simulink model "BlockV5"  (R2017a)
settings: Solver=VariableStepAuto  StartTime=0.0  StopTime=Tsim  FixedStep=Ts_compute  RelTol=1e-3
values from neighbouring files (symbols this model uses):
  A = [0 ur2 0;-ur2 0 ur1;0 0 0]    [Model_old.m]    (also in PIController.m)
  b = 0.1    [Model_old.m]
  C = eye(3)    [Model_old.m]    (also in PIController.m)
  g = 40    [Model_old.m]    (also in ModeloBase_OLD.m)
  J = 0.01    [Model_old.m]
  Kd = 0    [Model_old.m]
  Ke = 0.08    [Model_old.m]
  Ki = 10.0    (= 10)    [Model_old.m]
  Kp = 5.0    (= 5)    [Model_old.m]
  ksi = 0.6    [Model_old.m]    (also in ModeloBase_OLD.m = 0.3)
  L = 0.5    [Model_old.m]
  R = 1    [Model_old.m]
  Rv = var(noise.data)    [Model_old.m]
  Ts = 0.1    [Model_old.m]    (also in ModeloBase_OLD.m; PIController.m)
  Ts_sensor = 1/50    (= 0.02)    [Model_old.m]
undefined symbols (not defined in the file or in its folder): Ad, DiscIntNeverNeededParam, F_M, Rw, Ts_compute, Vd
libraries: simulink x26, cstblocks x6, simulink_extras x2
settings Model: PauseTimes=28  NumberOfSteps=10  Creator=davi2  LastModifiedBy=davi2

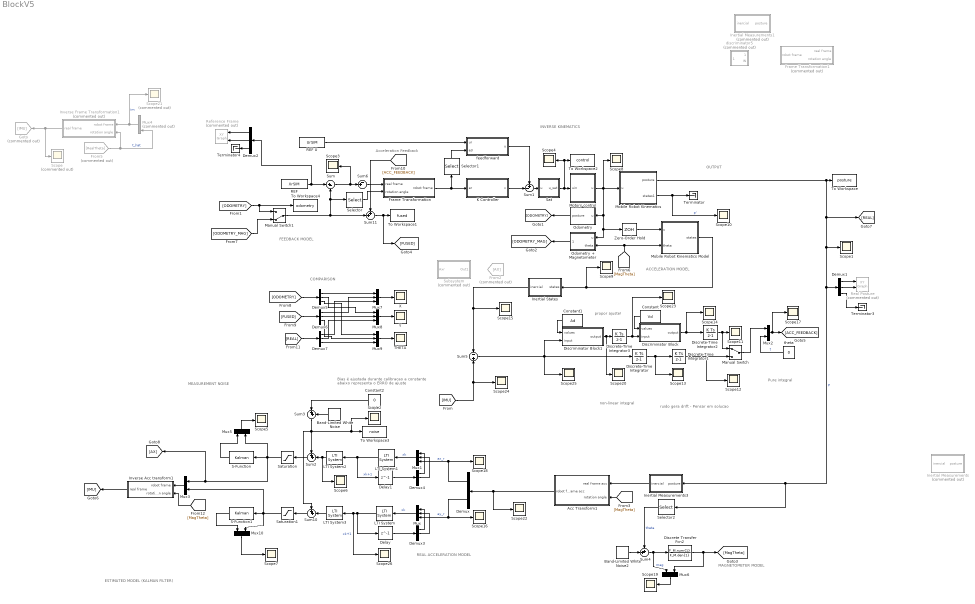
== system BlockV5 ==
  note: COMPARISON
  note: Bias é ajustada durante calibracao
      | a constante abaixo representa o ERRO de ajuste
  note: propor ajuste!
  note: Pure integral
  note: Acceleration Feedback
  note: ACCELERATION MODEL
  note: ruido gera drift - Pensar em solucao
  note: OUTPUT
  note: MEASUREMENT NOISE
  note: REAL ACCELERATION
      | MODEL
  note: INVERSE KINEMATICS
  note: MAGNETOMETER MODEL
  note: FEEDBACK MODEL
  note: ESTIMATED MODEL (KALMAN FILTER)
  note: non-linear integral
  Acc Transform1 : Subsystem
  Band-Limited White Noise : simulink/Sources/Band-Limited White Noise  Cov=0.00001  Ts=Ts_sensor  seed=[23341]
  Band-Limited White Noise2 : simulink/Sources/Band-Limited White Noise  Cov=0.00001  Ts=1/200  seed=[23341]
  Constant : Constant  Value=Vd
  Constant1 : Constant  Value=Ad
  Constant2 : Constant  Value=0
  Delay : Delay  DelayLength=1
  Delay1 : Delay  DelayLength=1
  Demux : Demux  Outputs=2
  Demux{1..7} (7 alike) : Demux  Outputs=3
  Discrete Transfer Fcn2 : DiscreteTransferFcn  Numerator=F_M.num{1}  Denominator=F_M.den{1}  SampleTime=Ts_sensor
  Discrete-Time Integrator{,1..3} (4 alike) : DiscreteIntegrator  InitialConditionSetting=State (most efficient)  SampleTime=Ts_sensor  ICPrevOutput=DiscIntNeverNeededParam  ICPrevScaledInput=DiscIntNeverNeededParam
  Discriminator Block : Subsystem
  Discriminator Block1 : Subsystem
  Frame Transformation : Subsystem
  Frame Transformation1 : Subsystem  Commented=on
  From2 : From  Commented=on  GotoTag=AX
  From5 : From  Commented=on  GotoTag=RealTheta
  Goto : Goto  Commented=on  GotoTag=IMU
  Inertial Measurements : Subsystem  Commented=on
  Inertial Measurements1 : Subsystem  Commented=on
  Inertial Measurements3 : Subsystem
  Inertial States : Subsystem
  Inverse Acc transform1 : Subsystem
  Inverse Frame Transformation1 : Subsystem  Commented=on
  K Controller : Subsystem
  LTI System : cstblocks/LTI System  sys=A  IC=[]
  LTI System1 : cstblocks/LTI System  sys=A  IC=[]
  LTI System2 : cstblocks/LTI System  sys=C  IC=[]
  LTI System3 : cstblocks/LTI System  sys=C  IC=[]
  Manual Switch : ManualSwitch
  Manual Switch1 : ManualSwitch  CurrentSetting=0
  Mobile Robot Kinematics : Subsystem
  Mobile Robot Kinematics Model : Subsystem
  Motors control : Subsystem
  Mux{,1,7..9} (5 alike) : Mux  Inputs=3
  Mux{2..3,5..6,10} (5 alike) : Mux  Inputs=2
  Mux4 : Mux  Commented=on  Inputs=3
  Odometry : Subsystem
  Odometry + Magnetometer : Subsystem
  REF : FromWorkspace  VariableName=XrSIM  SampleTime=Ts  OutputAfterFinalValue=Holding final value
  REF U : FromWorkspace  VariableName=UrSIM  SampleTime=Ts  OutputAfterFinalValue=Holding final value
  Real Posture : simulink/Sinks/XY Graph  Commented=on  xmin=0  xmax=3  ymin=-0.8  ymax=1.5  st=Ts
  Reference Frame : simulink/Sinks/XY Graph  Commented=on  xmin=0  xmax=2  ymin=0  ymax=1.5  st=Ts
  S-Function : S-Function  FunctionName=Kalman  Parameters=Ts_sensor,A,C,Rw,Rv  SFunctionDeploymentMode=off  EnableBusSupport=off
  S-Function1 : S-Function  FunctionName=Kalman  Parameters=Ts_sensor,A,C,Rw,Rv  SFunctionDeploymentMode=off  EnableBusSupport=off
  Sat : Subsystem
  Saturation : Saturate  UpperLimit=4*9.8  LowerLimit=-4*9.8
  Saturation1 : Saturate  UpperLimit=4*9.8  LowerLimit=-4*9.8
  Scope : Scope  Commented=on
  Scope{1..20,22..26} (25 alike) : Scope
  Scope21 : Scope  Commented=on
  Selector : Selector  InputPortWidth=3  IndexOptions=Index vector (dialog)  Indices=3  OutputSizes=1
  Selector1 : Selector  InputPortWidth=3  IndexOptions=Index vector (dialog)  Indices=3  OutputSizes=1
  Selector2 : Selector  InputPortWidth=3  IndexOptions=Index vector (dialog)  Indices=3  OutputSizes=1
  Subsystem : Subsystem  Commented=on
  Sum : Sum  Inputs=|+-
  Sum1 : Sum  Inputs=+-|
  Sum{2,4,10..11} (4 alike) : Sum  Inputs=++|
  Sum3 : Sum  Inputs=|++
  Sum5 : Sum  Inputs=-+
  Sum6 : Sum  Inputs=-+|
  THETA : Scope
  Terminator : Terminator
  Terminator3 : Terminator
  Terminator4 : Terminator
  To Workspace : ToWorkspace  VariableName=posture  SaveFormat=Timeseries  SampleTime=-1
  To Workspace1 : ToWorkspace  VariableName=fused  SaveFormat=Timeseries  SampleTime=-1
  To Workspace2 : ToWorkspace  VariableName=control  SaveFormat=Timeseries  SampleTime=-1
  To Workspace3 : ToWorkspace  VariableName=noise  SaveFormat=Timeseries  SampleTime=-1
  To Workspace4 : ToWorkspace  VariableName=odometry  SaveFormat=Timeseries  SampleTime=-1
  X : Scope
  Y : Scope
  Zero-Order Hold : ZeroOrderHold  SampleTime=Ts_sensor
  discriminator5 : Subsystem  Commented=on
  feedforward : Subsystem
  theta : Constant  Value=0
  wires:
  Sum/1 -> Sum6/2, Scope3/1
  Frame Transformation/1(robot frame) -> K Controller/1(er), Selector1/1
  REF U/1 -> feedforward/1(ur)
  Selector1/1 -> feedforward/2(e3)
  feedforward/1(u) -> Sum1/1
  K Controller/1(v) -> Sum1/2
  Motors control/1(u) -> Zero-Order Hold/1, Odometry + Magnetometer/1(u), Odometry/1(u), Mobile Robot Kinematics/1(u), Scope8/1
  Selector2/1 -> Sum4/1  "theta"
  Demux1/1 -> Real Posture/1
  Demux1/2 -> Real Posture/2
  REF/1 -> Demux2/1, Sum/1
  Odometry/1(posture) -> [ODOMETRY]
  Sum1/1 -> Sat/1(u)
  Sat/1(u_sat) -> Motors control/1(uin), Scope4/1, To Workspace2/1
  Demux1/3 -> Terminator3/1
  Band-Limited White Noise2/1 -> Sum4/2
  Sum4/1 -> Discrete Transfer Fcn2/1, Mux6/1  "mag"
  Discrete Transfer Fcn2/1 -> [MagTheta], Mux6/2
  Demux2/1 -> Reference Frame/1
  Demux2/2 -> Reference Frame/2
  Demux2/3 -> Terminator4/1
  LTI System/1 -> Scope26/1, LTI System3/1, Delay/1  "xk+1"
  Delay/1 -> Demux3/1
  Demux3/1 -> Mux/1
  Demux3/2 -> Mux/2
  Mux/1 -> LTI System/1  "xk"
  Demux4/2 -> Mux1/2
  Delay1/1 -> Demux4/1
  Demux4/1 -> Mux1/1
  LTI System1/1 -> Delay1/1, LTI System2/1  "xk+1"
  Mux1/1 -> LTI System1/1  "xk"
  Inverse Frame Transformation1/1(real frame) -> Goto/1, Scope/1
  From5/1 -> Mux4/3, Inverse Frame Transformation1/2(rotation angle)  "t_hat"
  LTI System3/1 -> Sum10/2
  Mux4/1 -> Scope21/1, Inverse Frame Transformation1/1(robot frame)  "im"
  Mobile Robot Kinematics/1(posture) -> [REAL], Selector2/1, Inertial Measurements3/1(posture), Demux1/1, Scope1/1, To Workspace/1  "P"
  Demux/1 -> Mux1/3, Scope18/1  "ax_r"
  Demux/2 -> Scope16/1, Mux/3  "ay_r"
  Inertial States/1(inercial) -> Sum5/1, Scope15/1
  Inertial Measurements3/1(inercial) -> Acc Transform1/1(real frame acc)
  Acc Transform1/1(robot frame acc) -> Scope22/1, Demux/1
  Sum6/1 -> Frame Transformation/1(real frame)
  theta/1 -> Mux2/2  "t"
  Mux2/1 -> Scope17/1, [ACC_FEEDBACK]
  LTI System2/1 -> Scope6/1, Sum2/2
  Sum11/1 -> [FUSED], To Workspace1/1
  Discrete-Time Integrator/1 -> Discrete-Time Integrator1/1, Scope13/1
  Mux5/1 -> Scope5/1
  Discrete-Time Integrator2/1 -> Scope11/1, Manual Switch/1
  Discrete-Time Integrator1/1 -> Manual Switch/2, Scope12/1
  Manual Switch/1 -> Mux2/1
  Discriminator Block/1(output) -> Discrete-Time Integrator2/1, Scope14/1
  Discriminator Block1/1(output) -> Scope20/1, Discrete-Time Integrator3/1
  Discrete-Time Integrator3/1 -> Discriminator Block/2(input), Scope23/1
  Constant1/1 -> Discriminator Block1/1(values)
  [ACC_FEEDBACK] -> Sum11/1
  Selector/1 -> Frame Transformation/2(rotation angle)
  [MagTheta] -> Acc Transform1/2(rotation angle)
  Odometry + Magnetometer/1(posture) -> [ODOMETRY_MAG]
  [MagTheta] -> Mobile Robot Kinematics Model/2("theta "), Odometry + Magnetometer/2(theta)
  [ODOMETRY] -> Manual Switch1/1, To Workspace4/1
  [ODOMETRY_MAG] -> Manual Switch1/2
  Manual Switch1/1 -> Selector/1, Sum/2, Sum11/2
  Mux6/1 -> Scope19/1
  [IMU] -> Scope24/1, Sum5/2
  [ODOMETRY] -> Demux5/1
  [FUSED] -> Demux6/1
  [REAL] -> Demux7/1
  Demux5/1 -> Mux7/1
  Demux6/1 -> Mux7/2
  Demux7/1 -> Mux7/3
  Mux7/1 -> X/1
  Demux5/2 -> Mux8/1
  Demux6/2 -> Mux8/2
  Demux7/2 -> Mux8/3
  Demux5/3 -> Mux9/1
  Demux6/3 -> Mux9/2
  Demux7/3 -> Mux9/3
  Mux8/1 -> Y/1
  Mux9/1 -> THETA/1
  Zero-Order Hold/1 -> Mobile Robot Kinematics Model/1(u)
  Mobile Robot Kinematics/2(states1) -> Scope10/1, Terminator/1  "p'"
  Mux3/1 -> Inverse Acc transform1/1(robot frame)
  [MagTheta] -> Inverse Acc transform1/2(rotation angle)
  Inverse Acc transform1/1(real frame) -> [IMU]
  Constant/1 -> Discriminator Block/1(values)
  Sum3/1 -> Sum10/1, Sum2/1, Scope2/1, To Workspace3/1
  Band-Limited White Noise/1 -> Sum3/2
  Constant2/1 -> Sum3/1
  Sum10/1 -> Saturation1/1
  Sum2/1 -> Saturation/1
  Sum5/1 -> Scope25/1, Discrete-Time Integrator/1, Discriminator Block1/2(input)
  Saturation1/1 -> Mux3/2, Mux10/2, S-Function1/1
  Saturation/1 -> [AX], Mux3/1, Mux5/2, S-Function/1
  S-Function1/1 -> Mux10/1
  Mux10/1 -> Scope7/1
  S-Function/1 -> Mux5/1
  Mobile Robot Kinematics Model/1(states) -> Scope9/1, Inertial States/1(states)

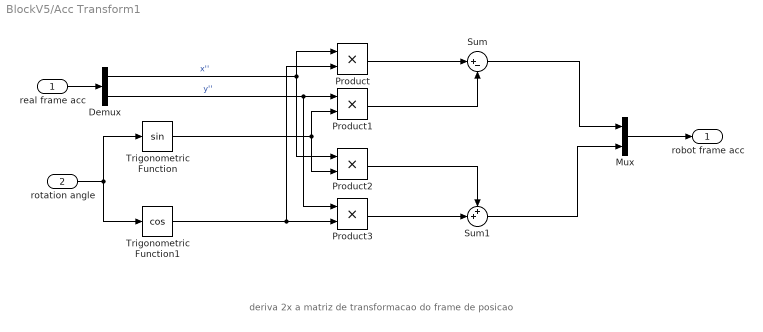
== system BlockV5/Acc Transform1 ==
  note: deriva 2x a matriz de transformacao do frame de posicao
  real frame acc : Inport
  rotation angle : Inport  Port=2
  Demux : Demux  Outputs=2
  Mux : Mux  Inputs=2
  Product{,1..3} (4 alike) : Product
  Sum : Sum  Inputs=|+-
  Sum1 : Sum  Inputs=++|
  Trigonometric Function : Trigonometry
  Trigonometric Function1 : Trigonometry  Operator=cos
  robot frame acc : Outport
  wires:
  rotation angle/1 -> Trigonometric Function/1, Trigonometric Function1/1
  Mux/1 -> robot frame acc/1
  real frame acc/1 -> Demux/1
  Demux/1 -> Product2/1, Product/1  "x''"
  Trigonometric Function1/1 -> Product/2, Product3/2
  Product/1 -> Sum/1
  Trigonometric Function/1 -> Product1/2, Product2/2
  Demux/2 -> Product3/1, Product1/1  "y''"
  Product1/1 -> Sum/2
  Sum/1 -> Mux/1
  Product3/1 -> Sum1/2
  Product2/1 -> Sum1/1
  Sum1/1 -> Mux/2

== system BlockV5/Discriminator Block ==
  values : Inport
  input : Inport  Port=2
  Demux : Demux  Outputs=2
  Mux : Mux  Inputs=2
  discriminator1 : Subsystem
  discriminator3 : Subsystem
  output : Outport
  wires:
  input/1 -> Demux/1
  Demux/1 -> discriminator3/2(IN)
  Demux/2 -> discriminator1/2(IN)
  Mux/1 -> output/1
  discriminator3/1(OUT) -> Mux/1
  discriminator1/1(OUT) -> Mux/2
  values/1 -> discriminator1/1(value), discriminator3/1(value)

== system BlockV5/Discriminator Block1 ==
  values : Inport
  input : Inport  Port=2
  Demux : Demux  Outputs=2
  Mux : Mux  Inputs=2
  discriminator1 : Subsystem
  discriminator3 : Subsystem
  output : Outport
  wires:
  input/1 -> Demux/1
  Demux/1 -> discriminator3/2(IN)
  Demux/2 -> discriminator1/2(IN)
  Mux/1 -> output/1
  discriminator3/1(OUT) -> Mux/1
  discriminator1/1(OUT) -> Mux/2
  values/1 -> discriminator1/1(value), discriminator3/1(value)

== system BlockV5/Frame Transformation ==
  real frame : Inport
  rotation angle : Inport  Port=2
  Mux : Mux  Inputs=2
  S-Function : S-Function  FunctionName=Real2Robot  Parameters=Ts  SFunctionDeploymentMode=off  EnableBusSupport=off
  robot frame : Outport
  wires:
  real frame/1 -> Mux/1
  rotation angle/1 -> Mux/2
  Mux/1 -> S-Function/1
  S-Function/1 -> robot frame/1

== system BlockV5/Frame Transformation1 ==
  real frame : Inport
  rotation angle : Inport  Port=2
  Mux : Mux  Inputs=2
  S-Function : S-Function  FunctionName=Real2Robot  Parameters=Ts_compute  SFunctionDeploymentMode=off  EnableBusSupport=off
  robot frame : Outport
  wires:
  real frame/1 -> Mux/1
  rotation angle/1 -> Mux/2
  Mux/1 -> S-Function/1
  S-Function/1 -> robot frame/1

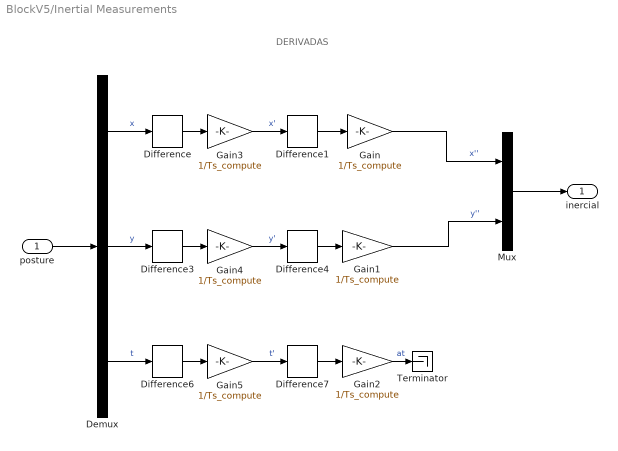
== system BlockV5/Inertial Measurements ==
  note: DERIVADAS
  posture : Inport
  Demux : Demux  Outputs=3
  Difference{,1,3..4,6..7} (6 alike) : simulink/Discrete/Difference  ICPrevInput=0.0  OutMin=[]  OutMax=[]  OutDataType=fixdt(1, 16)  OutScaling=2^-10  DoSatur=off
  Gain{,1..5} (6 alike) : Gain  Gain=1/Ts_compute
  Mux : Mux  Inputs=2
  Terminator : Terminator
  inercial : Outport
  wires:
  posture/1 -> Demux/1
  Demux/3 -> Difference6/1  "t"
  Demux/2 -> Difference3/1  "y"
  Demux/1 -> Difference/1  "x"
  Difference1/1 -> Gain/1
  Difference4/1 -> Gain1/1
  Difference7/1 -> Gain2/1
  Mux/1 -> inercial/1
  Gain2/1 -> Terminator/1  "at"
  Difference/1 -> Gain3/1
  Gain3/1 -> Difference1/1  "x'"
  Difference3/1 -> Gain4/1
  Gain4/1 -> Difference4/1  "y'"
  Difference6/1 -> Gain5/1
  Gain5/1 -> Difference7/1  "t'"
  Gain/1 -> Mux/1  "x''"
  Gain1/1 -> Mux/2  "y''"

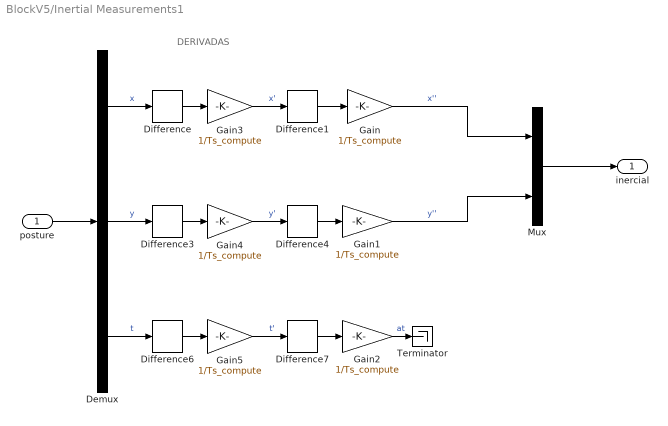
== system BlockV5/Inertial Measurements1 ==
  note: DERIVADAS
  posture : Inport
  Demux : Demux  Outputs=3
  Difference{,1,3..4,6..7} (6 alike) : simulink/Discrete/Difference  ICPrevInput=0.0  OutMin=[]  OutMax=[]  OutDataType=fixdt(1, 16)  OutScaling=2^-10  DoSatur=off
  Gain{,1..5} (6 alike) : Gain  Gain=1/Ts_compute
  Mux : Mux  Inputs=2
  Terminator : Terminator
  inercial : Outport
  wires:
  posture/1 -> Demux/1
  Demux/3 -> Difference6/1  "t"
  Demux/2 -> Difference3/1  "y"
  Demux/1 -> Difference/1  "x"
  Difference1/1 -> Gain/1
  Difference4/1 -> Gain1/1
  Difference7/1 -> Gain2/1
  Mux/1 -> inercial/1
  Gain2/1 -> Terminator/1  "at"
  Difference/1 -> Gain3/1
  Gain3/1 -> Difference1/1  "x'"
  Difference3/1 -> Gain4/1
  Gain4/1 -> Difference4/1  "y'"
  Difference6/1 -> Gain5/1
  Gain5/1 -> Difference7/1  "t'"
  Gain/1 -> Mux/1  "x''"
  Gain1/1 -> Mux/2  "y''"

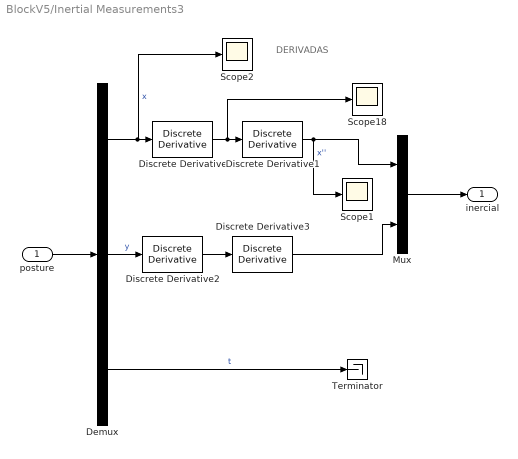
== system BlockV5/Inertial Measurements3 ==
  note: DERIVADAS
  posture : Inport
  Demux : Demux  Outputs=3
  Discrete Derivative{,1..3} (4 alike) : simulink/Discrete/Discrete Derivative  gainval=1.0  ICPrevScaledInput=0.0  OutMin=[]  OutMax=[]  OutDataType=fixdt(1, 16)  OutScaling=2^-10  DoSatur=off
  Mux : Mux  Inputs=2
  Scope1 : Scope
  Scope18 : Scope
  Scope2 : Scope
  Terminator : Terminator
  inercial : Outport
  wires:
  posture/1 -> Demux/1
  Demux/1 -> Discrete Derivative/1, Scope2/1  "x"
  Mux/1 -> inercial/1
  Discrete Derivative1/1 -> Scope1/1, Mux/1  "x''"
  Discrete Derivative/1 -> Scope18/1, Discrete Derivative1/1
  Demux/2 -> Discrete Derivative2/1  "y"
  Discrete Derivative2/1 -> Discrete Derivative3/1
  Discrete Derivative3/1 -> Mux/2
  Demux/3 -> Terminator/1  "t"

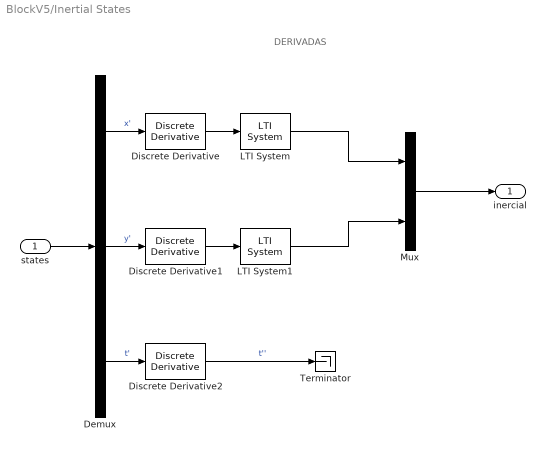
== system BlockV5/Inertial States ==
  note: DERIVADAS
  states : Inport
  Demux : Demux  Outputs=3
  Discrete Derivative : simulink/Discrete/Discrete Derivative  gainval=1.0  ICPrevScaledInput=0.0  OutMin=[]  OutMax=[]  OutDataType=fixdt(1, 16)  OutScaling=2^-10  DoSatur=off
  Discrete Derivative1 : simulink/Discrete/Discrete Derivative  gainval=1.0  ICPrevScaledInput=0.0  OutMin=[]  OutMax=[]  OutDataType=fixdt(1, 16)  OutScaling=2^-10  DoSatur=off
  Discrete Derivative2 : simulink/Discrete/Discrete Derivative  gainval=1.0  ICPrevScaledInput=0.0  OutMin=[]  OutMax=[]  OutDataType=fixdt(1, 16)  OutScaling=2^-10  DoSatur=off
  LTI System : cstblocks/LTI System  sys=MF  IC=[]
  LTI System1 : cstblocks/LTI System  sys=MF  IC=[]
  Mux : Mux  Inputs=2
  Terminator : Terminator
  inercial : Outport
  wires:
  states/1 -> Demux/1
  Mux/1 -> inercial/1
  Demux/3 -> Discrete Derivative2/1  "t'"
  Discrete Derivative2/1 -> Terminator/1  "t''"
  Demux/2 -> Discrete Derivative1/1  "y'"
  Demux/1 -> Discrete Derivative/1  "x'"
  Discrete Derivative1/1 -> LTI System1/1
  Discrete Derivative/1 -> LTI System/1
  LTI System/1 -> Mux/1
  LTI System1/1 -> Mux/2

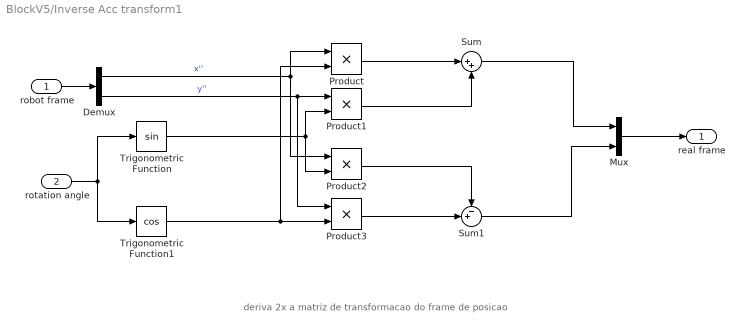
== system BlockV5/Inverse Acc transform1 ==
  note: deriva 2x a matriz de transformacao do frame de posicao
  robot frame : Inport
  rotation angle : Inport  Port=2
  Demux : Demux  Outputs=2
  Mux : Mux  Inputs=2
  Product{,1..3} (4 alike) : Product
  Sum : Sum  Inputs=|++
  Sum1 : Sum  Inputs=-+|
  Trigonometric Function : Trigonometry
  Trigonometric Function1 : Trigonometry  Operator=cos
  real frame : Outport
  wires:
  rotation angle/1 -> Trigonometric Function/1, Trigonometric Function1/1
  Mux/1 -> real frame/1
  robot frame/1 -> Demux/1
  Demux/1 -> Product2/1, Product/1  "x''"
  Trigonometric Function1/1 -> Product/2, Product3/2
  Product/1 -> Sum/1
  Trigonometric Function/1 -> Product1/2, Product2/2
  Demux/2 -> Product3/1, Product1/1  "y''"
  Product1/1 -> Sum/2
  Sum/1 -> Mux/1
  Product3/1 -> Sum1/2
  Product2/1 -> Sum1/1
  Sum1/1 -> Mux/2

== system BlockV5/Inverse Frame Transformation1 ==
  robot frame : Inport
  rotation angle : Inport  Port=2
  Mux : Mux  Inputs=2
  S-Function : S-Function  FunctionName=Robot2Real  Parameters=Ts  SFunctionDeploymentMode=off  EnableBusSupport=off
  real frame : Outport
  wires:
  S-Function/1 -> real frame/1
  Mux/1 -> S-Function/1
  rotation angle/1 -> Mux/2
  robot frame/1 -> Mux/1

== system BlockV5/K Controller ==
  er : Inport
  Constant : Constant  Value=ksi
  Constant1 : Constant  Value=g
  Mux : Mux  Inputs=5
  S-Function : S-Function  FunctionName=ControllerK  Parameters=Ts  SFunctionDeploymentMode=off  EnableBusSupport=off
  v : Outport
  wires:
  er/1 -> Mux/1
  [vr] -> Mux/2
  [wr] -> Mux/3
  Constant/1 -> Mux/4
  Constant1/1 -> Mux/5
  Mux/1 -> S-Function/1
  S-Function/1 -> v/1

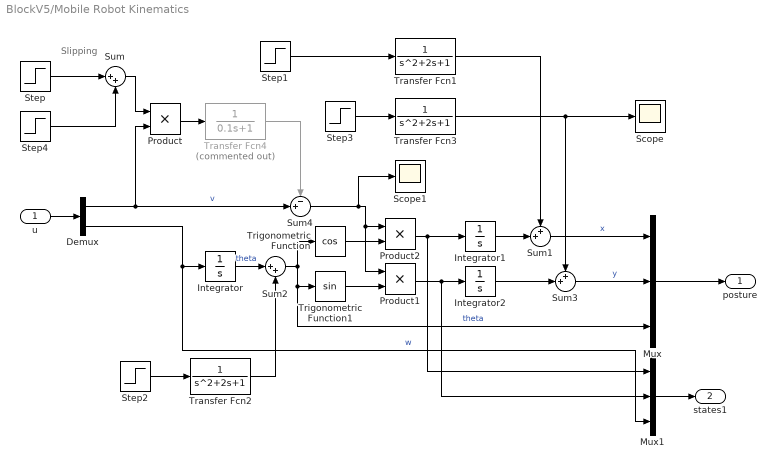
== system BlockV5/Mobile Robot Kinematics ==
  note: Slipping
  u : Inport
  Demux : Demux  Outputs=2
  Integrator : Integrator
  Integrator1 : Integrator
  Integrator2 : Integrator
  Mux : Mux  Inputs=3
  Mux1 : Mux  Inputs=3
  Product : Product
  Product1 : Product
  Product2 : Product
  Scope : Scope
  Scope1 : Scope
  Step : Step  Time=25  SampleTime=0
  Step1 : Step  Time=20  After=0  SampleTime=0
  Step2 : Step  Time=10  After=0  SampleTime=0
  Step3 : Step  Time=5  After=-1  SampleTime=0
  Step4 : Step  Time=27  After=-1  SampleTime=0
  Sum : Sum  Inputs=|++
  Sum1 : Sum  Inputs=++|
  Sum2 : Sum  Inputs=|++
  Sum3 : Sum  Inputs=++|
  Sum4 : Sum  Inputs=-+|
  Transfer Fcn1 : TransferFcn  Numerator=1
  Transfer Fcn2 : TransferFcn  Numerator=1
  Transfer Fcn3 : TransferFcn  Numerator=1
  Transfer Fcn4 : TransferFcn  Commented=on  Numerator=1  Denominator=[0.1 1]
  Trigonometric Function : Trigonometry  Operator=cos
  Trigonometric Function1 : Trigonometry
  posture : Outport
  states1 : Outport  Port=2
  wires:
  u/1 -> Demux/1
  Demux/2 -> Integrator/1, Mux1/3  "w"
  Trigonometric Function/1 -> Product2/2
  Demux/1 -> Sum4/2, Product/2  "v"
  Trigonometric Function1/1 -> Product1/2
  Mux/1 -> posture/1
  Step2/1 -> Transfer Fcn2/1
  Integrator/1 -> Sum2/1  "theta"
  Sum2/1 -> Mux/3, Trigonometric Function1/1, Trigonometric Function/1  "theta"
  Transfer Fcn2/1 -> Sum2/2
  Product1/1 -> Mux1/2, Integrator2/1
  Product2/1 -> Mux1/1, Integrator1/1
  Step1/1 -> Transfer Fcn1/1
  Step3/1 -> Transfer Fcn3/1
  Integrator1/1 -> Sum1/2
  Integrator2/1 -> Sum3/2
  Sum3/1 -> Mux/2  "y"
  Sum1/1 -> Mux/1  "x"
  Transfer Fcn3/1 -> Sum3/1, Scope/1
  Transfer Fcn1/1 -> Sum1/1
  Step/1 -> Sum/1
  Step4/1 -> Sum/2
  Sum/1 -> Product/1
  Sum4/1 -> Scope1/1, Product1/1, Product2/1
  Product/1 -> Transfer Fcn4/1
  Transfer Fcn4/1 -> Sum4/1
  Mux1/1 -> states1/1

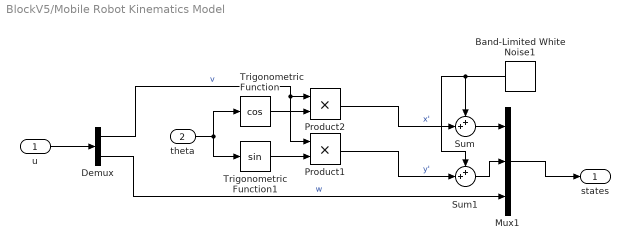
== system BlockV5/Mobile Robot Kinematics Model ==
  u : Inport
  "theta " : Inport  Port=2
  Band-Limited White Noise1 : simulink/Sources/Band-Limited White Noise  Cov=0.04^4  Ts=Ts  seed=[23341]
  Demux : Demux  Outputs=2
  Mux1 : Mux  Inputs=3
  Product1 : Product
  Product2 : Product
  Sum : Sum  Inputs=++|
  Sum1 : Sum  Inputs=++|
  Trigonometric Function : Trigonometry  Operator=cos
  Trigonometric Function1 : Trigonometry
  states : Outport
  wires:
  u/1 -> Demux/1
  Trigonometric Function/1 -> Product2/2
  Demux/1 -> Product1/1, Product2/1  "v"
  Trigonometric Function1/1 -> Product1/2
  Mux1/1 -> states/1
  "theta "/1 -> Trigonometric Function/1, Trigonometric Function1/1
  Demux/2 -> Mux1/3  "w"
  Product2/1 -> Sum/2  "x'"
  Product1/1 -> Sum1/2  "y'"
  Band-Limited White Noise1/1 -> Sum1/1, Sum/1
  Sum/1 -> Mux1/1
  Sum1/1 -> Mux1/2

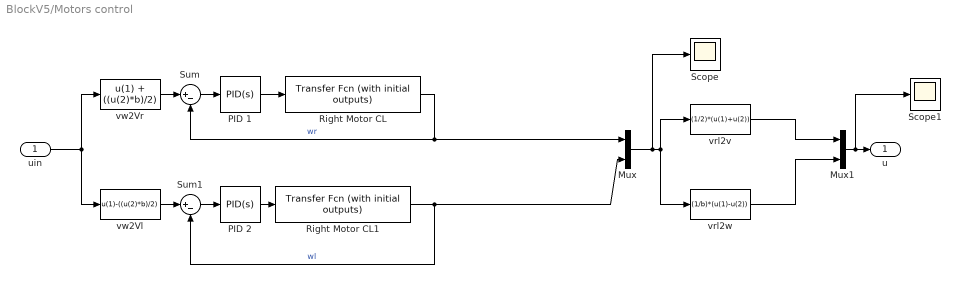
== system BlockV5/Motors control ==
  uin : Inport
  Mux : Mux  Inputs=2
  Mux1 : Mux  Inputs=2
  PID 1 : simulink/Continuous/PID Controller  Controller=PID  TimeDomain=Continuous-time  SampleTime=-1  IntegratorMethod=Forward Euler  FilterMethod=Forward Euler  Form=Parallel  UseFilter=on  ControllerParametersSource=internal  P=Kp  I=Ki  D=Kd  N=100  InitialConditionSource=internal  InitialConditionForIntegrator=0  InitialConditionForFilter=0  ExternalReset=none  LimitOutput=off  UpperSaturationLimit=inf  LowerSaturationLimit=-inf  LinearizeAsGain=on  AntiWindupMode=none  Kb=1  TrackingMode=off  Kt=1  PParamMin=[]  PParamMax=[]  IParamMin=[]  IParamMax=[]  DParamMin=[]  DParamMax=[]  NParamMin=[]  NParamMax=[]  KbParamMin=[]  KbParamMax=[]  KtParamMin=[]  KtParamMax=[]  POutMin=[]  POutMax=[]  IOutMin=[]  IOutMax=[]  DOutMin=[]  DOutMax=[]  NOutMin=[]  NOutMax=[]  KbOutMin=[]  KbOutMax=[]  KtOutMin=[]  KtOutMax=[]  IntegratorOutMin=[]  IntegratorOutMax=[]  FilterOutMin=[]  FilterOutMax=[]  SumOutMin=[]  SumOutMax=[]  SumI1OutMin=[]  SumI1OutMax=[]  SumI2OutMin=[]  SumI2OutMax=[]  SumI3OutMin=[]  SumI3OutMax=[]  SumDOutMin=[]  SumDOutMax=[]  SaturationOutMin=[]  SaturationOutMax=[]  IntegratorContinuousStateAttributes=''  IntegratorStateMustResolveToSignalObject=off  IntegratorRTWStateStorageClass=Auto  FilterContinuousStateAttributes=''  FilterStateMustResolveToSignalObject=off  FilterRTWStateStorageClass=Auto  DifferentiatorICPrevScaledInput=0  DifferentiatorOutMin=[]  DifferentiatorOutMax=[]  InitialConditionSetting=State (most efficient)
  PID 2 : simulink/Continuous/PID Controller  Controller=PID  TimeDomain=Continuous-time  SampleTime=-1  IntegratorMethod=Forward Euler  FilterMethod=Forward Euler  Form=Parallel  UseFilter=on  ControllerParametersSource=internal  P=Kp  I=Ki  D=Kd  N=100  InitialConditionSource=internal  InitialConditionForIntegrator=0  InitialConditionForFilter=0  ExternalReset=none  LimitOutput=off  UpperSaturationLimit=inf  LowerSaturationLimit=-inf  LinearizeAsGain=on  AntiWindupMode=none  Kb=1  TrackingMode=off  Kt=1  PParamMin=[]  PParamMax=[]  IParamMin=[]  IParamMax=[]  DParamMin=[]  DParamMax=[]  NParamMin=[]  NParamMax=[]  KbParamMin=[]  KbParamMax=[]  KtParamMin=[]  KtParamMax=[]  POutMin=[]  POutMax=[]  IOutMin=[]  IOutMax=[]  DOutMin=[]  DOutMax=[]  NOutMin=[]  NOutMax=[]  KbOutMin=[]  KbOutMax=[]  KtOutMin=[]  KtOutMax=[]  IntegratorOutMin=[]  IntegratorOutMax=[]  FilterOutMin=[]  FilterOutMax=[]  SumOutMin=[]  SumOutMax=[]  SumI1OutMin=[]  SumI1OutMax=[]  SumI2OutMin=[]  SumI2OutMax=[]  SumI3OutMin=[]  SumI3OutMax=[]  SumDOutMin=[]  SumDOutMax=[]  SaturationOutMin=[]  SaturationOutMax=[]  IntegratorContinuousStateAttributes=''  IntegratorStateMustResolveToSignalObject=off  IntegratorRTWStateStorageClass=Auto  FilterContinuousStateAttributes=''  FilterStateMustResolveToSignalObject=off  FilterRTWStateStorageClass=Auto  DifferentiatorICPrevScaledInput=0  DifferentiatorOutMin=[]  DifferentiatorOutMax=[]  InitialConditionSetting=State (most efficient)
  Right Motor CL : simulink_extras/Additional Linear/Transfer Fcn (with initial outputs)  N=[Ke]  D="[J*L  (J*R+b*L) (b*R+Ke^2)]"  Y0=0  U0=0
  Right Motor CL1 : simulink_extras/Additional Linear/Transfer Fcn (with initial outputs)  N=[Ke]  D="[J*L  (J*R+b*L) (b*R+Ke^2)]"  Y0=0  U0=0
  Scope : Scope
  Scope1 : Scope
  Sum : Sum  Inputs=|+-
  Sum1 : Sum  Inputs=|+-
  vrl2v : Fcn  Expr=(1/2)*(u(1)+u(2))
  vrl2w : Fcn  Expr=(1/b)*(u(1)-u(2))
  vw2Vl : Fcn  Expr=u(1)-((u(2)*b)/2)
  vw2Vr : Fcn  Expr=u(1) + ((u(2)*b)/2)
  u : Outport
  wires:
  vw2Vr/1 -> Sum/1
  Right Motor CL1/1 -> Mux/2, Sum1/2  "wl"
  vw2Vl/1 -> Sum1/1
  Sum1/1 -> PID 2/1
  PID 2/1 -> Right Motor CL1/1
  Sum/1 -> PID 1/1
  PID 1/1 -> Right Motor CL/1
  Right Motor CL/1 -> Mux/1, Sum/2  "wr"
  uin/1 -> vw2Vl/1, vw2Vr/1
  Mux/1 -> Scope/1, vrl2v/1, vrl2w/1
  Mux1/1 -> Scope1/1, u/1
  vrl2v/1 -> Mux1/1
  vrl2w/1 -> Mux1/2

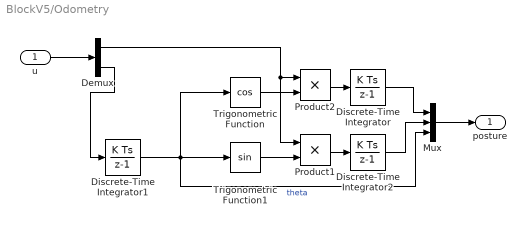
== system BlockV5/Odometry ==
  u : Inport
  Demux : Demux  Outputs=2
  Discrete-Time Integrator : DiscreteIntegrator  InitialConditionSetting=State (most efficient)  SampleTime=Ts  ICPrevOutput=DiscIntNeverNeededParam  ICPrevScaledInput=DiscIntNeverNeededParam
  Discrete-Time Integrator1 : DiscreteIntegrator  InitialConditionSetting=State (most efficient)  SampleTime=Ts  ICPrevOutput=DiscIntNeverNeededParam  ICPrevScaledInput=DiscIntNeverNeededParam
  Discrete-Time Integrator2 : DiscreteIntegrator  InitialConditionSetting=State (most efficient)  SampleTime=Ts  ICPrevOutput=DiscIntNeverNeededParam  ICPrevScaledInput=DiscIntNeverNeededParam
  Mux : Mux  Inputs=3
  Product1 : Product
  Product2 : Product
  Trigonometric Function : Trigonometry  Operator=cos
  Trigonometric Function1 : Trigonometry
  posture : Outport
  wires:
  u/1 -> Demux/1
  Demux/2 -> Discrete-Time Integrator1/1
  Trigonometric Function/1 -> Product2/2
  Demux/1 -> Product1/1, Product2/1
  Product2/1 -> Discrete-Time Integrator/1
  Trigonometric Function1/1 -> Product1/2
  Product1/1 -> Discrete-Time Integrator2/1
  Discrete-Time Integrator/1 -> Mux/1
  Discrete-Time Integrator2/1 -> Mux/2
  Mux/1 -> posture/1
  Discrete-Time Integrator1/1 -> Mux/3, Trigonometric Function1/1, Trigonometric Function/1  "theta"

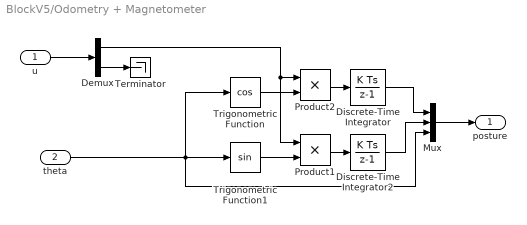
== system BlockV5/Odometry + Magnetometer ==
  u : Inport
  theta : Inport  Port=2
  Demux : Demux  Outputs=2
  Discrete-Time Integrator : DiscreteIntegrator  InitialConditionSetting=State (most efficient)  SampleTime=Ts  ICPrevOutput=DiscIntNeverNeededParam  ICPrevScaledInput=DiscIntNeverNeededParam
  Discrete-Time Integrator2 : DiscreteIntegrator  InitialConditionSetting=State (most efficient)  SampleTime=Ts  ICPrevOutput=DiscIntNeverNeededParam  ICPrevScaledInput=DiscIntNeverNeededParam
  Mux : Mux  Inputs=3
  Product1 : Product
  Product2 : Product
  Terminator : Terminator
  Trigonometric Function : Trigonometry  Operator=cos
  Trigonometric Function1 : Trigonometry
  posture : Outport
  wires:
  u/1 -> Demux/1
  Trigonometric Function/1 -> Product2/2
  Demux/1 -> Product1/1, Product2/1
  Product2/1 -> Discrete-Time Integrator/1
  Trigonometric Function1/1 -> Product1/2
  Product1/1 -> Discrete-Time Integrator2/1
  Discrete-Time Integrator/1 -> Mux/1
  Discrete-Time Integrator2/1 -> Mux/2
  Mux/1 -> posture/1
  Demux/2 -> Terminator/1
  theta/1 -> Mux/3, Trigonometric Function/1, Trigonometric Function1/1

== system BlockV5/Sat ==
  u : Inport
  Demux : Demux  Outputs=2
  Mux : Mux  Inputs=2
  Saturation : Saturate  UpperLimit=1  LowerLimit=0
  Saturation1 : Saturate  UpperLimit=1  LowerLimit=-1
  u_sat : Outport
  wires:
  Demux/2 -> Saturation1/1  "W"
  Demux/1 -> Saturation/1  "V"
  u/1 -> Demux/1
  Saturation/1 -> Mux/1
  Saturation1/1 -> Mux/2
  Mux/1 -> u_sat/1

== system BlockV5/Subsystem ==
  Axr : Inport
  Out1 : Outport

== system BlockV5/discriminator5 ==
  value : Inport
  IN : Inport  Port=2
  Abs : Abs
  If : If  NumInputs=2  IfExpression=u1 < u2
  If Action Subsystem : Subsystem  TreatAsAtomicUnit=on
  If Action Subsystem1 : Subsystem  TreatAsAtomicUnit=on
  Merge : Merge
  OUT : Outport
  wires:
  IN/1 -> If Action Subsystem1/1(In1), Abs/1
  Abs/1 -> If/1
  If/1 -> If Action Subsystem/Action
  If/2 -> If Action Subsystem1/Action
  If Action Subsystem/1(Out1) -> Merge/1
  If Action Subsystem1/1(Out1) -> Merge/2
  Merge/1 -> OUT/1
  value/1 -> If/2

== system BlockV5/feedforward ==
  ur : Inport
  e3 : Inport  Port=2
  Demux : Demux  Outputs=2
  Mux : Mux  Inputs=2
  Product : Product
  Trigonometric Function : Trigonometry  Operator=cos
  u : Outport
  tag scope: vr=global, wr=global
  wires:
  e3/1 -> Trigonometric Function/1
  ur/1 -> Demux/1
  Demux/1 -> [vr], Product/1
  Trigonometric Function/1 -> Product/2
  Product/1 -> Mux/1
  Demux/2 -> [wr], Mux/2
  Mux/1 -> u/1

== system BlockV5/Discriminator Block/discriminator1 ==
  value : Inport
  IN : Inport  Port=2
  Abs : Abs
  If : If  NumInputs=2  IfExpression=u1 < u2
  If Action Subsystem : Subsystem  TreatAsAtomicUnit=on
  If Action Subsystem1 : Subsystem  TreatAsAtomicUnit=on
  Merge : Merge
  OUT : Outport
  wires:
  IN/1 -> If Action Subsystem1/1(In1), Abs/1
  Abs/1 -> If/1
  If/1 -> If Action Subsystem/Action
  If/2 -> If Action Subsystem1/Action
  If Action Subsystem/1(Out1) -> Merge/1
  If Action Subsystem1/1(Out1) -> Merge/2
  Merge/1 -> OUT/1
  value/1 -> If/2

== system BlockV5/Discriminator Block/discriminator3 ==
  value : Inport
  IN : Inport  Port=2
  Abs : Abs
  If : If  NumInputs=2  IfExpression=u1 < u2
  If Action Subsystem : Subsystem  TreatAsAtomicUnit=on
  If Action Subsystem1 : Subsystem  TreatAsAtomicUnit=on
  Merge : Merge
  OUT : Outport
  wires:
  IN/1 -> If Action Subsystem1/1(In1), Abs/1
  Abs/1 -> If/1
  If/1 -> If Action Subsystem/Action
  If/2 -> If Action Subsystem1/Action
  If Action Subsystem/1(Out1) -> Merge/1
  If Action Subsystem1/1(Out1) -> Merge/2
  Merge/1 -> OUT/1
  value/1 -> If/2

== system BlockV5/Discriminator Block1/discriminator1 ==
  value : Inport
  IN : Inport  Port=2
  Abs : Abs  ZeroCross=off
  If : If  NumInputs=2  IfExpression=u1 < u2
  If Action Subsystem : Subsystem  TreatAsAtomicUnit=on
  If Action Subsystem1 : Subsystem  TreatAsAtomicUnit=on
  Merge : Merge
  OUT : Outport
  wires:
  IN/1 -> If Action Subsystem1/1(In1), Abs/1
  Abs/1 -> If/1
  If/1 -> If Action Subsystem/Action
  If/2 -> If Action Subsystem1/Action
  If Action Subsystem/1(Out1) -> Merge/1
  If Action Subsystem1/1(Out1) -> Merge/2
  Merge/1 -> OUT/1
  value/1 -> If/2

== system BlockV5/Discriminator Block1/discriminator3 ==
  value : Inport
  IN : Inport  Port=2
  Abs : Abs  ZeroCross=off
  If : If  NumInputs=2  IfExpression=u1 < u2
  If Action Subsystem : Subsystem  TreatAsAtomicUnit=on
  If Action Subsystem1 : Subsystem  TreatAsAtomicUnit=on
  Merge : Merge
  OUT : Outport
  wires:
  IN/1 -> If Action Subsystem1/1(In1), Abs/1
  Abs/1 -> If/1
  If/1 -> If Action Subsystem/Action
  If/2 -> If Action Subsystem1/Action
  If Action Subsystem/1(Out1) -> Merge/1
  If Action Subsystem1/1(Out1) -> Merge/2
  Merge/1 -> OUT/1
  value/1 -> If/2

== system BlockV5/discriminator5/If Action Subsystem ==
  Action Port : ActionPort  ActionType=then
  Constant : Constant  Value=0
  Out1 : Outport
  wires:
  Constant/1 -> Out1/1

== system BlockV5/discriminator5/If Action Subsystem1 ==
  In1 : Inport
  Action Port : ActionPort  ActionType=else
  Out1 : Outport
  wires:
  In1/1 -> Out1/1

== system BlockV5/Discriminator Block/discriminator1/If Action Subsystem ==
  Action Port : ActionPort  ActionType=then
  Constant : Constant  Value=0
  Out1 : Outport
  wires:
  Constant/1 -> Out1/1

== system BlockV5/Discriminator Block/discriminator1/If Action Subsystem1 ==
  In1 : Inport
  Action Port : ActionPort  ActionType=else
  Out1 : Outport
  wires:
  In1/1 -> Out1/1

== system BlockV5/Discriminator Block/discriminator3/If Action Subsystem ==
  Action Port : ActionPort  ActionType=then
  Constant : Constant  Value=0
  Out1 : Outport
  wires:
  Constant/1 -> Out1/1

== system BlockV5/Discriminator Block/discriminator3/If Action Subsystem1 ==
  In1 : Inport
  Action Port : ActionPort  ActionType=else
  Out1 : Outport
  wires:
  In1/1 -> Out1/1

== system BlockV5/Discriminator Block1/discriminator1/If Action Subsystem ==
  Action Port : ActionPort  ActionType=then
  Constant : Constant  Value=0
  Out1 : Outport
  wires:
  Constant/1 -> Out1/1

== system BlockV5/Discriminator Block1/discriminator1/If Action Subsystem1 ==
  In1 : Inport
  Action Port : ActionPort  ActionType=else
  Out1 : Outport
  wires:
  In1/1 -> Out1/1

== system BlockV5/Discriminator Block1/discriminator3/If Action Subsystem ==
  Action Port : ActionPort  ActionType=then
  Constant : Constant  Value=0
  Out1 : Outport
  wires:
  Constant/1 -> Out1/1

== system BlockV5/Discriminator Block1/discriminator3/If Action Subsystem1 ==
  In1 : Inport
  Action Port : ActionPort  ActionType=else
  Out1 : Outport
  wires:
  In1/1 -> Out1/1
